simulink model "svpwm_v3"  (R2017a)
settings: Solver=FixedStepAuto  StartTime=0  StopTime=100e-3  FixedStep=1/252000  MaxStep=1e-4  RelTol=1e-4
values from neighbouring files (symbols this model uses):
  Amp = 600    [svpwm_param_v1.m]
  fs = 4e3    (= 4000)    [svpwm_param_v1.m]
  Ts = (1/fs)    (= 0.00025)    [svpwm_param_v1.m]
  Vdc = 700    [svpwm_param_v1.m]
  Vref = 400    [svpwm_param_v1.m]
libraries: powerlib x16, simulink x2, simulink_extras x1
settings Model: Creator=Shuvangkar  LastModifiedBy=Shuvangkar

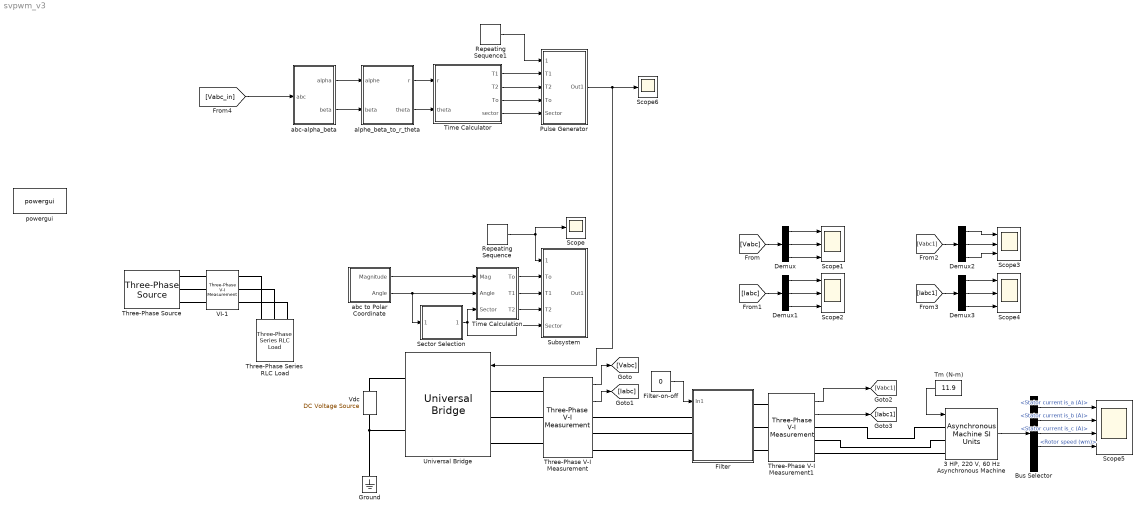
== system svpwm_v3 ==
  "3 HP, 220 V, 60 Hz Asynchronous Machine" : powerlib/Machines/Asynchronous Machine SI Units  RotorType=Squirrel-cage  PresetModel=No  MechanicalLoad=Torque Tm  ShowDetailedParameters=on  ReferenceFrame=Stationary  Units=SI  MeasurementBus=off  NominalParameters=[ 3*746, 220, 60 ]  Stator="[ 0.435  2*2.0e-3 ]"  Rotor="[ 0.816  2.0e-3 ]"  Cage1=[ 0.022 0.226/377]  Cage2=[ 0.022 0.226/377]  Lm=69.31e-3  Mechanical="[ 0.089  0  2 ]"  PolePairs=2  InitialConditions=[0.044533 0 11.138 11.138 11.138 -39.6 -159.6 80.4]  SimulateSaturation=off  Saturation=[0 0;0 0]  LoadFlowParameters=2000  TsPowergui=0  TsBlock=-1  IterativeModel=Trapezoidal non iterative  IterativeDiscreteModel=Trapezoidal non iterative  Pmec=0
  Bus Selector : BusSelector  OutputSignals=Stator measurements.Stator current is_a (A),Stator measurements.Stator current is_b (A),Stator measurements.Stator current is_c (A),Mechanical.Rotor speed (wm),Mechanical.Electromagnetic torque Te (N*m)
  Demux{,1..3} (4 alike) : Demux  Outputs=3
  Filter : Subsystem
  Filter-on-off : Constant  Value=0
  Ground : powerlib/Elements/Ground  LConnTagsString=a
  Pulse Generator : Subsystem
  Repeating Sequence : simulink/Sources/Repeating Sequence  rep_seq_t=[0 1/2 1]*(1/fs)  rep_seq_y=[0 1 0]
  Repeating Sequence1 : simulink/Sources/Repeating Sequence  rep_seq_t=[0 1/2 1]*(1/fs)  rep_seq_y=[0 1 0]
  Scope : Scope
  Scope{1..4} (4 alike) : Scope  NumInputPorts=3
  Scope5 : Scope  NumInputPorts=4
  Scope6 : Scope
  Sector Selection : Subsystem
  Subsystem : Subsystem
  Three-Phase Series RLC Load : powerlib/Elements/Three-Phase Series RLC Load  LConnTagsString=A|B|C  Configuration=Y (grounded)  NominalVoltage=400  Vabc=[1e3 1e3 1e3]  Vabcp=[1e3 1e3 1e3]  NominalFrequency=50  UnbalancedPower=off  ActivePower=10e3  InductivePower=100  CapacitivePower=100  Pabc=[10e3 9e3 11e3]  QLabc=[100 90 110]  QCabc=[100 90 110]  Pabcp=[10e3 9e3 11e3]  QLabcp=[100 90 110]  QCabcp=[100 90 110]  Measurements=None  LoadType=constant Z
  Three-Phase V-I Measurement : powerlib/Measurements/Three-Phase V-I Measurement  VoltageMeasurement=phase-to-phase  SetLabelV=off  LabelV=Vabc  Vpu=off  VpuLL=off  CurrentMeasurement=yes  SetLabelI=off  LabelI=Iabc  Ipu=off  Pbase=100e6  Vbase=500e3  OutputType=Complex  PhasorSimulation=off  PSBequivalent=0
  Three-Phase V-I Measurement1 : powerlib/Measurements/Three-Phase V-I Measurement  VoltageMeasurement=phase-to-ground  SetLabelV=off  LabelV=Vabc  Vpu=off  VpuLL=off  CurrentMeasurement=yes  SetLabelI=off  LabelI=Iabc  Ipu=off  Pbase=100e6  Vbase=500e3  OutputType=Complex  PhasorSimulation=off  PSBequivalent=0
  Three-Phase Source : powerlib/Electrical Sources/Three-Phase Source  InternalConnection=Yg  VoltagePhases=off  Voltage=400  PhaseAngle=0  Voltage_phases=[25e3 25e3 25e3]/sqrt(3)  PhaseAngles_phases=[0 -120 +120]  Frequency=50  NonIdealSource=on  SpecifyImpedance=off  Resistance=0.8929  Inductance=16.58e-3  ShortCircuitLevel=100e6  BaseVoltage=25e3  XRratio=7  BusType=swing  Pref=10e3  Qref=0  Prefabc=[10e3, 10e3, 10e3]  Qrefabc=[0, 0, 0]  Qmin=-inf  Qmax=inf
  Time Calculation : Subsystem
  Time Calculator : Subsystem
  Tm (N-m) : Constant  Value=11.9
  Universal Bridge : powerlib/Power Electronics/Universal Bridge  Arms=3  SnubberResistance=1e5  SnubberCapacitance=inf  Device=MOSFET / Diodes  Ron=1e-3  Lon=0  ForwardVoltages="[  0  0  ]"  ForwardVoltage=0  GTOparameters=[ 10e-6 , 20e-6 ]  IGBTparameters=[ 1e-6 , 2e-6 ]  Measurements=None  Measurements_2=None  converterType=Rectifier
  VI-1 : powerlib/Measurements/Three-Phase V-I Measurement  VoltageMeasurement=phase-to-ground  SetLabelV=on  LabelV=Vabc_in  Vpu=off  VpuLL=off  CurrentMeasurement=yes  SetLabelI=on  LabelI=Iabc_in  Ipu=off  Pbase=100e6  Vbase=500e3  OutputType=Complex  PhasorSimulation=off  PSBequivalent=0
  Vdc : powerlib/Electrical Sources/DC Voltage Source  Amplitude=Amp  Measurements=None
  abc to Polar Coordinate : Subsystem
  abc-alpha_beta : Subsystem
  alphe_beta_to_r_theta : Subsystem
  powergui : powerlib/powergui  Priority=1  SimulationMode=Discrete  SampleTime=1/252000  frequency=60  Iterations=50  frequencyindice=60  Pbase=100e6  ErrMax=1e-4  UnitsV=kV  UnitsW=MW  buscounter=0  FunctionMessages=off  echomessages=off  EnableUseOfTLC=off  CurrentSourceSwitches=off  DisableSnubberDevices=off  DisableRonSwitches=off  DisableVfSwitches=off  DisplayEquations=off  SolverType=Tustin/Backward Euler (TBE)  Interpol=off  ExternalGateDelay=off  methode=off  Ts=100  x0status=blocks  SPID=off  SwTol=0  HookPort=off  RestoreLinks=warning  ResistiveCurrentMeasurement=off  Frange=[0:2:500]  Ylog=off  Xlog=on  ShowGrid=off  save=off  variable=ZData  structure=0  ZoomFFT=off  StartTime=0.0  cycles=1  DisplayStyle=1  fundamental=60  FreqAxis=off  MaxFrequency=1000  frequencyindicesteady=1  RmsSteady=1  display=off
  wires:
  abc to Polar Coordinate/2(Angle) -> Sector Selection/1(Angle), Time Calculation/2(Angle)
  abc to Polar Coordinate/1(Magnitude) -> Time Calculation/1(Mag)
  Sector Selection/1(Sector) -> Subsystem/5(Sector), Time Calculation/3(Sector)
  Repeating Sequence/1 -> Scope/1, Subsystem/1(Sequence)
  Time Calculation/1(To) -> Subsystem/2(To)
  Time Calculation/3(T2) -> Subsystem/4(T2)
  Time Calculation/2(T1) -> Subsystem/3(T1)
  Filter-on-off/1 -> Filter/1(In1)
  Three-Phase V-I Measurement/1 -> [Vabc]
  Three-Phase V-I Measurement/2 -> [Iabc]
  [Vabc] -> Demux/1
  Demux/1 -> Scope1/1
  Demux/2 -> Scope1/2
  Demux/3 -> Scope1/3
  Demux1/2 -> Scope2/2
  [Iabc] -> Demux1/1
  Demux1/1 -> Scope2/1
  Demux1/3 -> Scope2/3
  Three-Phase V-I Measurement1/2 -> [Iabc1]
  Three-Phase V-I Measurement1/1 -> [Vabc1]
  [Iabc1] -> Demux3/1
  Demux2/3 -> Scope3/3
  Demux3/3 -> Scope4/3
  Demux2/2 -> Scope3/2
  Demux2/1 -> Scope3/1
  [Vabc1] -> Demux2/1
  Demux3/2 -> Scope4/2
  Demux3/1 -> Scope4/1
  Tm (N-m)/1 -> "3 HP, 220 V, 60 Hz Asynchronous Machine"/1
  "3 HP, 220 V, 60 Hz Asynchronous Machine"/1 -> Bus Selector/1
  Bus Selector/1 -> Scope5/1  "<Stator current is_a (A)>"
  Bus Selector/2 -> Scope5/2  "<Stator current is_b (A)>"
  Bus Selector/3 -> Scope5/3  "<Stator current is_c (A)>"
  Bus Selector/4 -> Scope5/4  "<Rotor speed (wm)>"
  [Vabc_in] -> abc-alpha_beta/1(abc)
  abc-alpha_beta/1(alpha) -> alphe_beta_to_r_theta/1(alphe)
  abc-alpha_beta/2(beta) -> alphe_beta_to_r_theta/2(beta)
  alphe_beta_to_r_theta/1(r) -> Time Calculator/1(r)
  alphe_beta_to_r_theta/2(theta) -> Time Calculator/2(theta)
  Repeating Sequence1/1 -> Pulse Generator/1(Sequence)
  Pulse Generator/1(Out1) -> Universal Bridge/1, Scope6/1
  Time Calculator/1(T1) -> Pulse Generator/2(T1)
  Time Calculator/2(T2) -> Pulse Generator/3(T2)
  Time Calculator/3(To) -> Pulse Generator/4(To)
  Time Calculator/4(sector) -> Pulse Generator/5(Sector)
  connections:
  Universal Bridge/RConn2 -- Vdc/LConn1 -- Ground/LConn1
  Vdc/RConn1 -- Universal Bridge/RConn1
  Three-Phase V-I Measurement/LConn1 -- Universal Bridge/LConn1
  Three-Phase V-I Measurement/LConn2 -- Universal Bridge/LConn2
  Three-Phase V-I Measurement/LConn3 -- Universal Bridge/LConn3
  Three-Phase V-I Measurement/RConn1 -- Filter/LConn1
  Three-Phase V-I Measurement/RConn2 -- Filter/LConn2
  Three-Phase V-I Measurement/RConn3 -- Filter/LConn3
  Filter/RConn1 -- Three-Phase V-I Measurement1/LConn1
  Filter/RConn2 -- Three-Phase V-I Measurement1/LConn2
  Filter/RConn3 -- Three-Phase V-I Measurement1/LConn3
  "3 HP, 220 V, 60 Hz Asynchronous Machine"/LConn1 -- Three-Phase V-I Measurement1/RConn1
  "3 HP, 220 V, 60 Hz Asynchronous Machine"/LConn2 -- Three-Phase V-I Measurement1/RConn2
  "3 HP, 220 V, 60 Hz Asynchronous Machine"/LConn3 -- Three-Phase V-I Measurement1/RConn3
  VI-1/LConn1 -- Three-Phase Source/RConn1
  VI-1/LConn2 -- Three-Phase Source/RConn2
  VI-1/LConn3 -- Three-Phase Source/RConn3
  VI-1/RConn1 -- Three-Phase Series RLC Load/LConn1
  VI-1/RConn2 -- Three-Phase Series RLC Load/LConn2
  VI-1/RConn3 -- Three-Phase Series RLC Load/LConn3

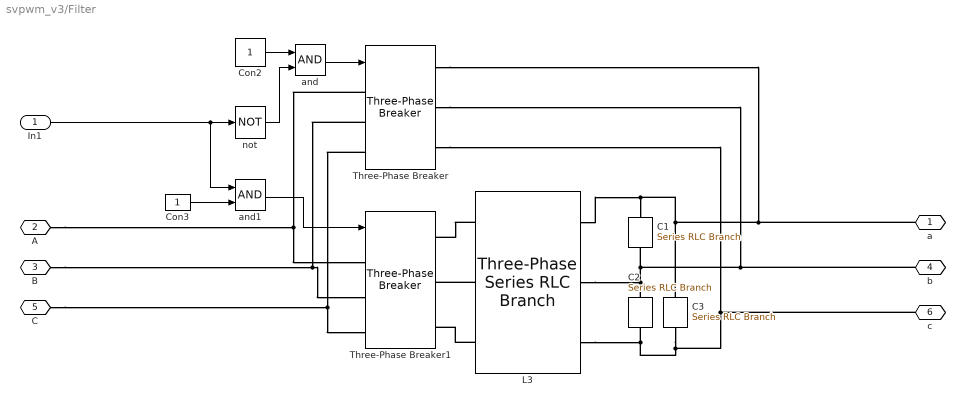
== system svpwm_v3/Filter ==
  In1 : Inport
  C1 : powerlib/Elements/Series RLC Branch  LConnTagsString=__new0  RConnTagsString=__new0  BranchType=C  Resistance=1  Inductance=1e-3  SetiL0=off  InitialCurrent=0  Capacitance=5e-6  Setx0=off  InitialVoltage=0  Measurements=None
  C2 : powerlib/Elements/Series RLC Branch  LConnTagsString=__new0  RConnTagsString=__new0  BranchType=C  Resistance=1  Inductance=1e-3  SetiL0=off  InitialCurrent=0  Capacitance=5e-6  Setx0=off  InitialVoltage=0  Measurements=None
  C3 : powerlib/Elements/Series RLC Branch  LConnTagsString=__new0  RConnTagsString=__new0  BranchType=C  Resistance=1  Inductance=1e-3  SetiL0=off  InitialCurrent=0  Capacitance=5e-6  Setx0=off  InitialVoltage=0  Measurements=None
  Con2 : Constant
  Con3 : Constant
  L3 : powerlib/Elements/Three-Phase Series RLC Branch  LConnTagsString=A|B|C  RConnTagsString=A|B|C  BranchType=L  Resistance=1  Inductance=10e-3  Capacitance=1e-6  Measurements=None
  Three-Phase Breaker : powerlib/Elements/Three-Phase Breaker  InitialState=open  SwitchA=on  SwitchB=on  SwitchC=on  SwitchTimes="[1/60  5/60]"  External=on  BreakerResistance=1e-6  SnubberResistance=1e6  SnubberCapacitance=inf  Measurements=None
  Three-Phase Breaker1 : powerlib/Elements/Three-Phase Breaker  InitialState=open  SwitchA=on  SwitchB=on  SwitchC=on  SwitchTimes="[1/60  5/60]"  External=on  BreakerResistance=0.01  SnubberResistance=1e6  SnubberCapacitance=inf  Measurements=None
  and : Logic  AllPortsSameDT=off  OutDataTypeStr=boolean
  and1 : Logic  AllPortsSameDT=off  OutDataTypeStr=boolean
  not : Logic  Operator=NOT  AllPortsSameDT=off  OutDataTypeStr=boolean
  a : PMIOPort  Port=1  Side=Right
  A : PMIOPort  Port=2  Side=Left
  B : PMIOPort  Port=3  Side=Left
  b : PMIOPort  Port=4  Side=Right
  C : PMIOPort  Port=5  Side=Left
  c : PMIOPort  Port=6  Side=Right
  wires:
  Con3/1 -> and1/2
  and/1 -> Three-Phase Breaker/1
  and1/1 -> Three-Phase Breaker1/1
  Con2/1 -> and/1
  In1/1 -> and1/1, not/1
  not/1 -> and/2
  connections:
  Three-Phase Breaker/LConn2 -- B/RConn1 -- Three-Phase Breaker1/LConn2
  L3/LConn1 -- Three-Phase Breaker1/RConn1
  L3/LConn2 -- Three-Phase Breaker1/RConn2
  L3/LConn3 -- Three-Phase Breaker1/RConn3
  Three-Phase Breaker/LConn1 -- A/RConn1 -- Three-Phase Breaker1/LConn1
  L3/RConn2 -- b/RConn1 -- Three-Phase Breaker/RConn2 -- C1/RConn1 -- C2/LConn1
  L3/RConn3 -- c/RConn1 -- Three-Phase Breaker/RConn3 -- C3/LConn1 -- C2/RConn1
  Three-Phase Breaker/LConn3 -- C/RConn1 -- Three-Phase Breaker1/LConn3
  C3/RConn1 -- a/RConn1 -- Three-Phase Breaker/RConn1 -- C1/LConn1 -- L3/RConn1

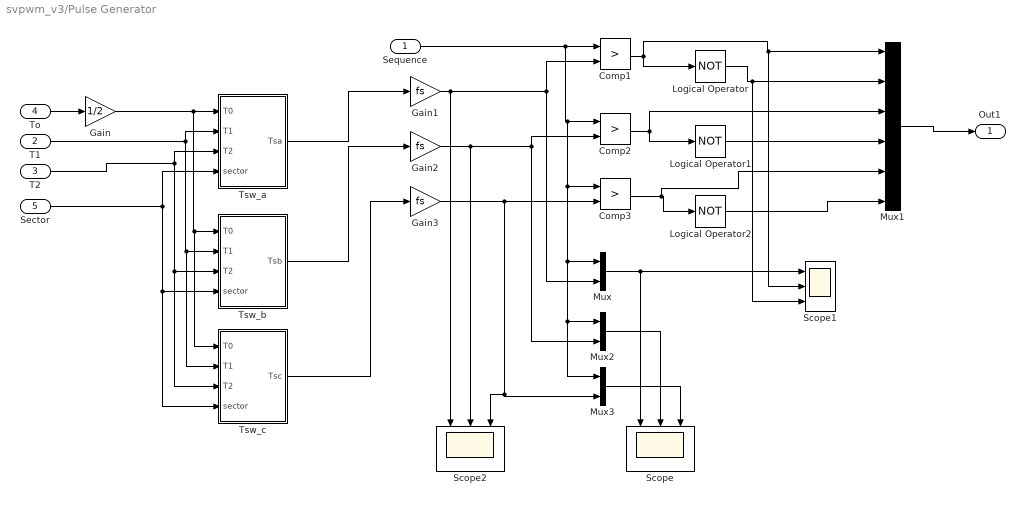
== system svpwm_v3/Pulse Generator ==
  Sequence : Inport
  T1 : Inport  Port=2
  T2 : Inport  Port=3
  To : Inport  Port=4
  Sector : Inport  Port=5
  Comp1 : RelationalOperator  Operator=>  OutDataTypeStr=boolean  RndMeth=Simplest
  Comp2 : RelationalOperator  Operator=>  OutDataTypeStr=boolean  RndMeth=Simplest
  Comp3 : RelationalOperator  Operator=>  OutDataTypeStr=boolean  RndMeth=Simplest
  Gain : Gain  Gain=1/2
  Gain1 : Gain  Gain=fs
  Gain2 : Gain  Gain=fs
  Gain3 : Gain  Gain=fs
  Logical Operator : Logic  Operator=NOT  AllPortsSameDT=off  OutDataTypeStr=boolean
  Logical Operator1 : Logic  Operator=NOT  AllPortsSameDT=off  OutDataTypeStr=boolean
  Logical Operator2 : Logic  Operator=NOT  AllPortsSameDT=off  OutDataTypeStr=boolean
  Mux : Mux  Inputs=2
  Mux1 : Mux  Inputs=6
  Mux2 : Mux  Inputs=2
  Mux3 : Mux  Inputs=2
  Scope : Scope  NumInputPorts=3
  Scope1 : Scope  NumInputPorts=3
  Scope2 : Scope  NumInputPorts=3
  Tsw_a : MATLAB Function  TreatAsAtomicUnit=on
  Tsw_b : MATLAB Function  TreatAsAtomicUnit=on
  Tsw_c : MATLAB Function  TreatAsAtomicUnit=on
  Out1 : Outport
  wires:
  Sector/1 -> Tsw_c/4(sector), Tsw_b/4(sector), Tsw_a/4(sector)
  To/1 -> Gain/1
  Gain/1 -> Tsw_c/1(T0), Tsw_b/1(T0), Tsw_a/1(T0)
  T2/1 -> Tsw_c/3(T2), Tsw_b/3(T2), Tsw_a/3(T2)
  T1/1 -> Tsw_c/2(T1), Tsw_b/2(T1), Tsw_a/2(T1)
  Mux1/1 -> Out1/1
  Gain2/1 -> Scope2/2, Mux2/2, Comp2/2
  Logical Operator2/1 -> Mux1/6
  Gain3/1 -> Scope2/3, Mux3/2, Comp3/2
  Comp1/1 -> Logical Operator/1, Scope1/2, Mux1/1
  Comp3/1 -> Mux1/5, Logical Operator2/1
  Sequence/1 -> Mux3/1, Mux2/1, Mux/1, Comp3/1, Comp2/1, Comp1/1
  Comp2/1 -> Logical Operator1/1, Mux1/3
  Logical Operator/1 -> Scope1/3, Mux1/2
  Logical Operator1/1 -> Mux1/4
  Gain1/1 -> Scope2/1, Mux/2, Comp1/2
  Tsw_a/1(Tsa) -> Gain1/1
  Tsw_b/1(Tsb) -> Gain2/1
  Tsw_c/1(Tsc) -> Gain3/1
  Mux2/1 -> Scope/2
  Mux/1 -> Scope1/1, Scope/1
  Mux3/1 -> Scope/3

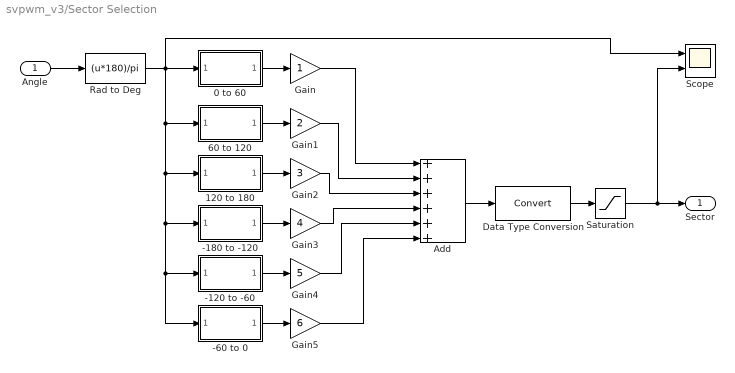
== system svpwm_v3/Sector Selection ==
  Angle : Inport
  -120 to -60 : Subsystem
  -180 to -120 : Subsystem
  -60 to 0 : Subsystem
  0 to 60 : Subsystem
  120 to 180 : Subsystem
  60 to 120 : Subsystem
  Add : Sum  Inputs=++++++
  Data Type Conversion : DataTypeConversion
  Gain : Gain
  Gain1 : Gain  Gain=2
  Gain2 : Gain  Gain=3
  Gain3 : Gain  Gain=4
  Gain4 : Gain  Gain=5
  Gain5 : Gain  Gain=6
  Rad to Deg : Fcn  Expr=(u*180)/pi
  Saturation : Saturate  UpperLimit=6  LowerLimit=1
  Scope : Scope  NumInputPorts=2
  Sector : Outport
  wires:
  Rad to Deg/1 -> Scope/1, -120 to -60/1(Angle), -60 to 0/1(Angle), -180 to -120/1(Angle), 120 to 180/1(Angle), 60 to 120/1(Angle), 0 to 60/1(Angle)
  Angle/1 -> Rad to Deg/1
  Gain4/1 -> Add/5
  0 to 60/1(sector) -> Gain/1
  60 to 120/1(sector) -> Gain1/1
  -120 to -60/1(sector) -> Gain4/1
  -180 to -120/1(sector) -> Gain3/1
  Gain5/1 -> Add/6
  -60 to 0/1(sector) -> Gain5/1
  Gain/1 -> Add/1
  120 to 180/1(sector) -> Gain2/1
  Gain1/1 -> Add/2
  Gain2/1 -> Add/3
  Gain3/1 -> Add/4
  Saturation/1 -> Scope/2, Sector/1
  Add/1 -> Data Type Conversion/1
  Data Type Conversion/1 -> Saturation/1

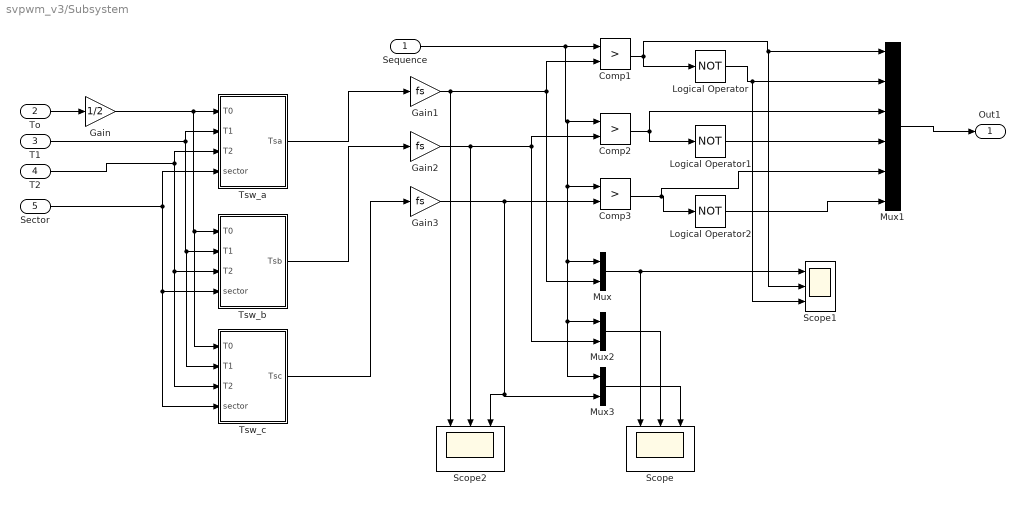
== system svpwm_v3/Subsystem ==
  Sequence : Inport
  To : Inport  Port=2
  T1 : Inport  Port=3
  T2 : Inport  Port=4
  Sector : Inport  Port=5
  Comp1 : RelationalOperator  Operator=>  OutDataTypeStr=boolean  RndMeth=Simplest
  Comp2 : RelationalOperator  Operator=>  OutDataTypeStr=boolean  RndMeth=Simplest
  Comp3 : RelationalOperator  Operator=>  OutDataTypeStr=boolean  RndMeth=Simplest
  Gain : Gain  Gain=1/2
  Gain1 : Gain  Gain=fs
  Gain2 : Gain  Gain=fs
  Gain3 : Gain  Gain=fs
  Logical Operator : Logic  Operator=NOT  AllPortsSameDT=off  OutDataTypeStr=boolean
  Logical Operator1 : Logic  Operator=NOT  AllPortsSameDT=off  OutDataTypeStr=boolean
  Logical Operator2 : Logic  Operator=NOT  AllPortsSameDT=off  OutDataTypeStr=boolean
  Mux : Mux  Inputs=2
  Mux1 : Mux  Inputs=6
  Mux2 : Mux  Inputs=2
  Mux3 : Mux  Inputs=2
  Scope : Scope  NumInputPorts=3
  Scope1 : Scope  NumInputPorts=3
  Scope2 : Scope  NumInputPorts=3
  Tsw_a : MATLAB Function  TreatAsAtomicUnit=on
  Tsw_b : MATLAB Function  TreatAsAtomicUnit=on
  Tsw_c : MATLAB Function  TreatAsAtomicUnit=on
  Out1 : Outport
  wires:
  Sector/1 -> Tsw_c/4(sector), Tsw_b/4(sector), Tsw_a/4(sector)
  To/1 -> Gain/1
  Gain/1 -> Tsw_c/1(T0), Tsw_b/1(T0), Tsw_a/1(T0)
  T2/1 -> Tsw_c/3(T2), Tsw_b/3(T2), Tsw_a/3(T2)
  T1/1 -> Tsw_c/2(T1), Tsw_b/2(T1), Tsw_a/2(T1)
  Mux1/1 -> Out1/1
  Gain2/1 -> Scope2/2, Mux2/2, Comp2/2
  Logical Operator2/1 -> Mux1/6
  Gain3/1 -> Scope2/3, Mux3/2, Comp3/2
  Comp1/1 -> Logical Operator/1, Scope1/2, Mux1/1
  Comp3/1 -> Mux1/5, Logical Operator2/1
  Sequence/1 -> Mux3/1, Mux2/1, Mux/1, Comp3/1, Comp2/1, Comp1/1
  Comp2/1 -> Logical Operator1/1, Mux1/3
  Logical Operator/1 -> Scope1/3, Mux1/2
  Logical Operator1/1 -> Mux1/4
  Gain1/1 -> Scope2/1, Mux/2, Comp1/2
  Tsw_a/1(Tsa) -> Gain1/1
  Tsw_b/1(Tsb) -> Gain2/1
  Tsw_c/1(Tsc) -> Gain3/1
  Mux2/1 -> Scope/2
  Mux/1 -> Scope1/1, Scope/1
  Mux3/1 -> Scope/3

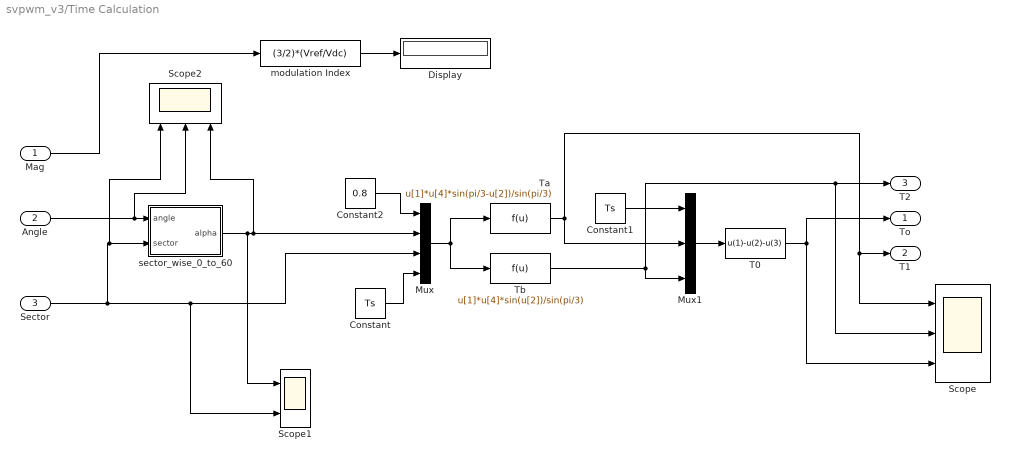
== system svpwm_v3/Time Calculation ==
  Mag : Inport
  Angle : Inport  Port=2
  Sector : Inport  Port=3
  Constant : Constant  Value=Ts
  Constant1 : Constant  Value=Ts
  Constant2 : Constant  Value=0.8
  Display : Display
  Mux : Mux
  Mux1 : Mux  Inputs=3
  Scope : Scope  NumInputPorts=3
  Scope1 : Scope  NumInputPorts=2
  Scope2 : Scope  NumInputPorts=3
  T0 : Fcn  Expr=u(1)-u(2)-u(3)
  Ta : Fcn  Expr=u[1]*u[4]*sin(pi/3-u[2])/sin(pi/3)
  Tb : Fcn  Expr=u[1]*u[4]*sin(u[2])/sin(pi/3)
  modulation Index : Fcn  Expr=(3/2)*(Vref/Vdc)
  "sector_wise_0_to_60 " : MATLAB Function  TreatAsAtomicUnit=on
  To : Outport
  T1 : Outport  Port=2
  T2 : Outport  Port=3
  wires:
  Mux1/1 -> T0/1
  modulation Index/1 -> Display/1
  Constant/1 -> Mux/4
  Ta/1 -> Scope/1, T1/1, Mux1/2
  T0/1 -> Scope/3, To/1
  Tb/1 -> Scope/2, T2/1, Mux1/3
  Mux/1 -> Tb/1, Ta/1
  Sector/1 -> Scope2/1, "sector_wise_0_to_60 "/2(sector), Scope1/2, Mux/3
  Constant1/1 -> Mux1/1
  Mag/1 -> modulation Index/1
  Constant2/1 -> Mux/1
  "sector_wise_0_to_60 "/1(alpha) -> Scope1/1, Scope2/3, Mux/2
  Angle/1 -> Scope2/2, "sector_wise_0_to_60 "/1(angle)

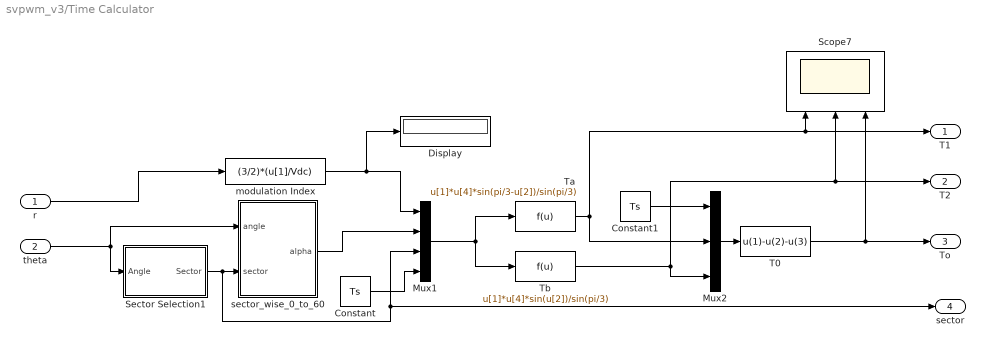
== system svpwm_v3/Time Calculator ==
  r : Inport
  theta : Inport  Port=2
  Constant : Constant  Value=Ts
  Constant1 : Constant  Value=Ts
  Display : Display
  Mux1 : Mux
  Mux2 : Mux  Inputs=3
  Scope7 : Scope  NumInputPorts=3
  Sector Selection1 : Subsystem
  T0 : Fcn  Expr=u(1)-u(2)-u(3)
  Ta : Fcn  Expr=u[1]*u[4]*sin(pi/3-u[2])/sin(pi/3)
  Tb : Fcn  Expr=u[1]*u[4]*sin(u[2])/sin(pi/3)
  modulation Index : Fcn  Expr=(3/2)*(u[1]/Vdc)
  "sector_wise_0_to_60 " : MATLAB Function  TreatAsAtomicUnit=on
  T1 : Outport
  T2 : Outport  Port=2
  To : Outport  Port=3
  sector : Outport  Port=4
  wires:
  Sector Selection1/1(Sector) -> sector/1, Mux1/3, "sector_wise_0_to_60 "/2(sector)
  r/1 -> modulation Index/1
  theta/1 -> Sector Selection1/1(Angle), "sector_wise_0_to_60 "/1(angle)
  modulation Index/1 -> Display/1, Mux1/1
  Constant1/1 -> Mux2/1
  Tb/1 -> T2/1, Scope7/2, Mux2/3
  Ta/1 -> T1/1, Scope7/1, Mux2/2
  Mux1/1 -> Tb/1, Ta/1
  Mux2/1 -> T0/1
  Constant/1 -> Mux1/4
  T0/1 -> To/1, Scope7/3
  "sector_wise_0_to_60 "/1(alpha) -> Mux1/2

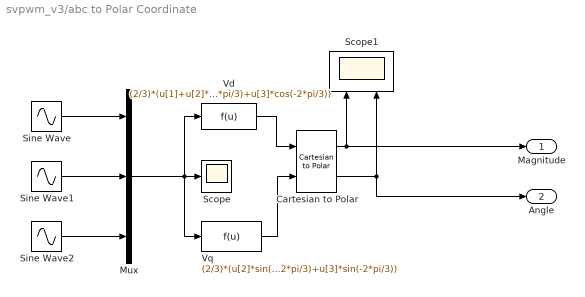
== system svpwm_v3/abc to Polar Coordinate ==
  Cartesian to Polar : simulink_extras/Transformations/Cartesian to Polar
      settings: SourceProductName=Simulink
  Mux : Mux  Inputs=3
  Scope : Scope
  Scope1 : Scope  NumInputPorts=2
  Sine Wave : Sin  Amplitude=Amp  Frequency=2*pi*50  SampleTime=0
  Sine Wave1 : Sin  Amplitude=Amp  Frequency=2*pi*50  Phase=2*pi/3  SampleTime=0
  Sine Wave2 : Sin  Amplitude=Amp  Frequency=2*pi*50  Phase=4*pi/3  SampleTime=0
  Vd : Fcn  Expr=(2/3)*(u[1]+u[2]*cos(2*pi/3)+u[3]*cos(-2*pi/3))
  Vq : Fcn  Expr=(2/3)*(u[2]*sin(2*pi/3)+u[3]*sin(-2*pi/3))
  Magnitude : Outport
  Angle : Outport  Port=2
  wires:
  Mux/1 -> Vq/1, Vd/1, Scope/1
  Cartesian to Polar/2 -> Angle/1, Scope1/2
  Cartesian to Polar/1 -> Magnitude/1, Scope1/1
  Vq/1 -> Cartesian to Polar/2
  Vd/1 -> Cartesian to Polar/1
  Sine Wave/1 -> Mux/1
  Sine Wave1/1 -> Mux/2
  Sine Wave2/1 -> Mux/3

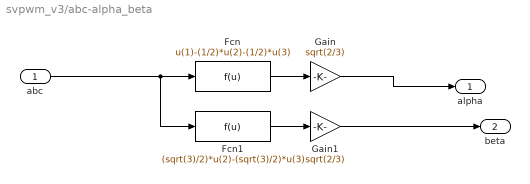
== system svpwm_v3/abc-alpha_beta ==
  abc : Inport
  Fcn : Fcn  Expr=u(1)-(1/2)*u(2)-(1/2)*u(3)
  Fcn1 : Fcn  Expr=(sqrt(3)/2)*u(2)-(sqrt(3)/2)*u(3)
  Gain : Gain  Gain=sqrt(2/3)
  Gain1 : Gain  Gain=sqrt(2/3)
  alpha : Outport
  beta : Outport  Port=2
  wires:
  abc/1 -> Fcn1/1, Fcn/1
  Gain/1 -> alpha/1
  Fcn/1 -> Gain/1
  Fcn1/1 -> Gain1/1
  Gain1/1 -> beta/1

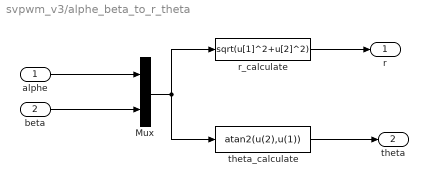
== system svpwm_v3/alphe_beta_to_r_theta ==
  alphe : Inport
  beta : Inport  Port=2
  Mux : Mux  Inputs=2
  r_calculate : Fcn  Expr=sqrt(u[1]^2+u[2]^2)
  theta_calculate : Fcn  Expr=atan2(u(2),u(1))
  r : Outport
  theta : Outport  Port=2
  wires:
  Mux/1 -> theta_calculate/1, r_calculate/1
  theta_calculate/1 -> theta/1
  r_calculate/1 -> r/1
  alphe/1 -> Mux/1
  beta/1 -> Mux/2

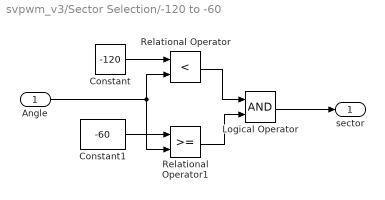
== system svpwm_v3/Sector Selection/-120 to -60 ==
  Angle : Inport
  Constant : Constant  Value=-120
  Constant1 : Constant  Value=-60
  Logical Operator : Logic  AllPortsSameDT=off  OutDataTypeStr=boolean
  Relational Operator : RelationalOperator  Operator=<  OutDataTypeStr=boolean  RndMeth=Simplest
  Relational Operator1 : RelationalOperator  OutDataTypeStr=boolean  RndMeth=Simplest
  sector : Outport
  wires:
  Relational Operator/1 -> Logical Operator/1
  Constant1/1 -> Relational Operator1/1
  Constant/1 -> Relational Operator/1
  Relational Operator1/1 -> Logical Operator/2
  Angle/1 -> Relational Operator/2, Relational Operator1/2
  Logical Operator/1 -> sector/1

== system svpwm_v3/Sector Selection/-180 to -120 ==
  Angle : Inport
  Constant : Constant  Value=-180
  Constant1 : Constant  Value=-120
  Logical Operator : Logic  AllPortsSameDT=off  OutDataTypeStr=boolean
  Relational Operator : RelationalOperator  Operator=<  OutDataTypeStr=boolean  RndMeth=Simplest
  Relational Operator1 : RelationalOperator  OutDataTypeStr=boolean  RndMeth=Simplest
  sector : Outport
  wires:
  Relational Operator/1 -> Logical Operator/1
  Constant1/1 -> Relational Operator1/1
  Constant/1 -> Relational Operator/1
  Relational Operator1/1 -> Logical Operator/2
  Angle/1 -> Relational Operator/2, Relational Operator1/2
  Logical Operator/1 -> sector/1

== system svpwm_v3/Sector Selection/-60 to 0 ==
  Angle : Inport
  Constant : Constant  Value=-60
  Constant1 : Constant  Value=0
  Logical Operator : Logic  AllPortsSameDT=off  OutDataTypeStr=boolean
  Relational Operator : RelationalOperator  Operator=<  OutDataTypeStr=boolean  RndMeth=Simplest
  Relational Operator1 : RelationalOperator  OutDataTypeStr=boolean  RndMeth=Simplest
  sector : Outport
  wires:
  Relational Operator/1 -> Logical Operator/1
  Constant1/1 -> Relational Operator1/1
  Constant/1 -> Relational Operator/1
  Relational Operator1/1 -> Logical Operator/2
  Angle/1 -> Relational Operator/2, Relational Operator1/2
  Logical Operator/1 -> sector/1

== system svpwm_v3/Sector Selection/0 to 60 ==
  Angle : Inport
  Constant : Constant  Value=0
  Constant1 : Constant  Value=60
  Logical Operator : Logic  AllPortsSameDT=off  OutDataTypeStr=boolean
  Relational Operator : RelationalOperator  Operator=<  OutDataTypeStr=boolean  RndMeth=Simplest
  Relational Operator1 : RelationalOperator  OutDataTypeStr=boolean  RndMeth=Simplest
  sector : Outport
  wires:
  Relational Operator/1 -> Logical Operator/1
  Constant1/1 -> Relational Operator1/1
  Constant/1 -> Relational Operator/1
  Relational Operator1/1 -> Logical Operator/2
  Angle/1 -> Relational Operator1/2, Relational Operator/2
  Logical Operator/1 -> sector/1

== system svpwm_v3/Sector Selection/120 to 180 ==
  Angle : Inport
  Constant : Constant  Value=120
  Constant1 : Constant  Value=180
  Logical Operator : Logic  AllPortsSameDT=off  OutDataTypeStr=boolean
  Relational Operator : RelationalOperator  Operator=<  OutDataTypeStr=boolean  RndMeth=Simplest
  Relational Operator1 : RelationalOperator  OutDataTypeStr=boolean  RndMeth=Simplest
  sector : Outport
  wires:
  Relational Operator/1 -> Logical Operator/1
  Constant1/1 -> Relational Operator1/1
  Constant/1 -> Relational Operator/1
  Relational Operator1/1 -> Logical Operator/2
  Angle/1 -> Relational Operator/2, Relational Operator1/2
  Logical Operator/1 -> sector/1

== system svpwm_v3/Sector Selection/60 to 120 ==
  Angle : Inport
  Constant : Constant  Value=60
  Constant1 : Constant  Value=120
  Logical Operator : Logic  AllPortsSameDT=off  OutDataTypeStr=boolean
  Relational Operator : RelationalOperator  Operator=<  OutDataTypeStr=boolean  RndMeth=Simplest
  Relational Operator1 : RelationalOperator  OutDataTypeStr=boolean  RndMeth=Simplest
  sector : Outport
  wires:
  Relational Operator/1 -> Logical Operator/1
  Constant1/1 -> Relational Operator1/1
  Constant/1 -> Relational Operator/1
  Relational Operator1/1 -> Logical Operator/2
  Angle/1 -> Relational Operator/2, Relational Operator1/2
  Logical Operator/1 -> sector/1

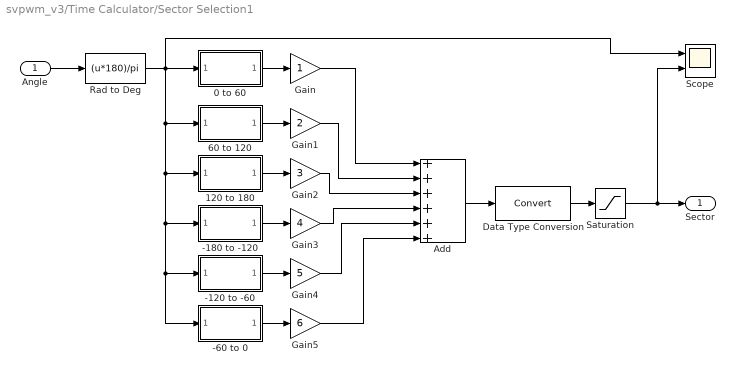
== system svpwm_v3/Time Calculator/Sector Selection1 ==
  Angle : Inport
  -120 to -60 : Subsystem
  -180 to -120 : Subsystem
  -60 to 0 : Subsystem
  0 to 60 : Subsystem
  120 to 180 : Subsystem
  60 to 120 : Subsystem
  Add : Sum  Inputs=++++++
  Data Type Conversion : DataTypeConversion
  Gain : Gain
  Gain1 : Gain  Gain=2
  Gain2 : Gain  Gain=3
  Gain3 : Gain  Gain=4
  Gain4 : Gain  Gain=5
  Gain5 : Gain  Gain=6
  Rad to Deg : Fcn  Expr=(u*180)/pi
  Saturation : Saturate  UpperLimit=6  LowerLimit=1
  Scope : Scope  NumInputPorts=2
  Sector : Outport
  wires:
  Rad to Deg/1 -> Scope/1, -120 to -60/1(Angle), -60 to 0/1(Angle), -180 to -120/1(Angle), 120 to 180/1(Angle), 60 to 120/1(Angle), 0 to 60/1(Angle)
  Angle/1 -> Rad to Deg/1
  Gain4/1 -> Add/5
  0 to 60/1(sector) -> Gain/1
  60 to 120/1(sector) -> Gain1/1
  -120 to -60/1(sector) -> Gain4/1
  -180 to -120/1(sector) -> Gain3/1
  Gain5/1 -> Add/6
  -60 to 0/1(sector) -> Gain5/1
  Gain/1 -> Add/1
  120 to 180/1(sector) -> Gain2/1
  Gain1/1 -> Add/2
  Gain2/1 -> Add/3
  Gain3/1 -> Add/4
  Saturation/1 -> Scope/2, Sector/1
  Add/1 -> Data Type Conversion/1
  Data Type Conversion/1 -> Saturation/1

== system svpwm_v3/Time Calculator/Sector Selection1/-120 to -60 ==
  Angle : Inport
  Constant : Constant  Value=-120
  Constant1 : Constant  Value=-60
  Logical Operator : Logic  AllPortsSameDT=off  OutDataTypeStr=boolean
  Relational Operator : RelationalOperator  Operator=<  OutDataTypeStr=boolean  RndMeth=Simplest
  Relational Operator1 : RelationalOperator  OutDataTypeStr=boolean  RndMeth=Simplest
  sector : Outport
  wires:
  Relational Operator/1 -> Logical Operator/1
  Constant1/1 -> Relational Operator1/1
  Constant/1 -> Relational Operator/1
  Relational Operator1/1 -> Logical Operator/2
  Angle/1 -> Relational Operator/2, Relational Operator1/2
  Logical Operator/1 -> sector/1

== system svpwm_v3/Time Calculator/Sector Selection1/-180 to -120 ==
  Angle : Inport
  Constant : Constant  Value=-180
  Constant1 : Constant  Value=-120
  Logical Operator : Logic  AllPortsSameDT=off  OutDataTypeStr=boolean
  Relational Operator : RelationalOperator  Operator=<  OutDataTypeStr=boolean  RndMeth=Simplest
  Relational Operator1 : RelationalOperator  OutDataTypeStr=boolean  RndMeth=Simplest
  sector : Outport
  wires:
  Relational Operator/1 -> Logical Operator/1
  Constant1/1 -> Relational Operator1/1
  Constant/1 -> Relational Operator/1
  Relational Operator1/1 -> Logical Operator/2
  Angle/1 -> Relational Operator/2, Relational Operator1/2
  Logical Operator/1 -> sector/1

== system svpwm_v3/Time Calculator/Sector Selection1/-60 to 0 ==
  Angle : Inport
  Constant : Constant  Value=-60
  Constant1 : Constant  Value=0
  Logical Operator : Logic  AllPortsSameDT=off  OutDataTypeStr=boolean
  Relational Operator : RelationalOperator  Operator=<  OutDataTypeStr=boolean  RndMeth=Simplest
  Relational Operator1 : RelationalOperator  OutDataTypeStr=boolean  RndMeth=Simplest
  sector : Outport
  wires:
  Relational Operator/1 -> Logical Operator/1
  Constant1/1 -> Relational Operator1/1
  Constant/1 -> Relational Operator/1
  Relational Operator1/1 -> Logical Operator/2
  Angle/1 -> Relational Operator/2, Relational Operator1/2
  Logical Operator/1 -> sector/1

== system svpwm_v3/Time Calculator/Sector Selection1/0 to 60 ==
  Angle : Inport
  Constant : Constant  Value=0
  Constant1 : Constant  Value=60
  Logical Operator : Logic  AllPortsSameDT=off  OutDataTypeStr=boolean
  Relational Operator : RelationalOperator  Operator=<  OutDataTypeStr=boolean  RndMeth=Simplest
  Relational Operator1 : RelationalOperator  OutDataTypeStr=boolean  RndMeth=Simplest
  sector : Outport
  wires:
  Relational Operator/1 -> Logical Operator/1
  Constant1/1 -> Relational Operator1/1
  Constant/1 -> Relational Operator/1
  Relational Operator1/1 -> Logical Operator/2
  Angle/1 -> Relational Operator1/2, Relational Operator/2
  Logical Operator/1 -> sector/1

== system svpwm_v3/Time Calculator/Sector Selection1/120 to 180 ==
  Angle : Inport
  Constant : Constant  Value=120
  Constant1 : Constant  Value=180
  Logical Operator : Logic  AllPortsSameDT=off  OutDataTypeStr=boolean
  Relational Operator : RelationalOperator  Operator=<  OutDataTypeStr=boolean  RndMeth=Simplest
  Relational Operator1 : RelationalOperator  OutDataTypeStr=boolean  RndMeth=Simplest
  sector : Outport
  wires:
  Relational Operator/1 -> Logical Operator/1
  Constant1/1 -> Relational Operator1/1
  Constant/1 -> Relational Operator/1
  Relational Operator1/1 -> Logical Operator/2
  Angle/1 -> Relational Operator/2, Relational Operator1/2
  Logical Operator/1 -> sector/1

== system svpwm_v3/Time Calculator/Sector Selection1/60 to 120 ==
  Angle : Inport
  Constant : Constant  Value=60
  Constant1 : Constant  Value=120
  Logical Operator : Logic  AllPortsSameDT=off  OutDataTypeStr=boolean
  Relational Operator : RelationalOperator  Operator=<  OutDataTypeStr=boolean  RndMeth=Simplest
  Relational Operator1 : RelationalOperator  OutDataTypeStr=boolean  RndMeth=Simplest
  sector : Outport
  wires:
  Relational Operator/1 -> Logical Operator/1
  Constant1/1 -> Relational Operator1/1
  Constant/1 -> Relational Operator/1
  Relational Operator1/1 -> Logical Operator/2
  Angle/1 -> Relational Operator/2, Relational Operator1/2
  Logical Operator/1 -> sector/1

== matlab function svpwm_v3/Subsystem/Tsw_a ==
  data: T0 input; Tsa output; T1 input; T2 input; sector input
function Tsa = fcn(T0,T1,T2,sector)
if(sector==1)
    Tsa = T0+T1+T2;  
elseif(sector==2)
    Tsa = T1+T0;  
elseif(sector==3)
    Tsa = T0;  
elseif(sector==4)
    Tsa = T0;  
elseif(sector==5)
    Tsa = T2+T0;  
else(sector==6)
    Tsa = T1+T2+T0;
end

== matlab function svpwm_v3/Time Calculation/sector_wise_0_to_60  ==
  data: angle input; alpha output; sector input
function alpha = fcn(angle,sector)
alpha = 0;
if (sector==1)
    alpha = angle;
elseif (sector==2)
    alpha = angle-pi/3;
elseif (sector == 3)
    alpha = angle- (2*pi/3);
elseif (sector==4)
    alpha = angle+pi;
elseif (sector==5)
    alpha = angle+(2*pi/3)
else 
    alpha = angle+pi/3;
end

== matlab function svpwm_v3/Subsystem/Tsw_b ==
  data: T0 input; Tsb output; T1 input; T2 input; sector input
function Tsb = fcn(T0,T1,T2,sector)
if(sector==1)
    Tsb = T2+T0;  
elseif(sector==2)
    Tsb = T0+T1+T2; 
elseif(sector==3)
    Tsb = T0+T1+T2;  
elseif(sector==4)
    Tsb = T0+T1;  
elseif(sector==5)
    Tsb = T0;  
else(sector==6)
    Tsb = T0;
end

== matlab function svpwm_v3/Subsystem/Tsw_c ==
  data: T0 input; Tsc output; T1 input; T2 input; sector input
function Tsc = fcn(T0,T1,T2,sector)
if(sector==1)
    Tsc = T0;  
elseif(sector==2)
    Tsc = T0;  
elseif(sector==3)
    Tsc = T0+T2;  
elseif(sector==4)
    Tsc = T0+T1+T2;  
elseif(sector==5)
    Tsc = T0+T1+T2;  
else(sector==6)
    Tsc = T0+T1;
end

== matlab function svpwm_v3/Time Calculator/sector_wise_0_to_60  ==
  data: angle input; alpha output; sector input
function alpha = fcn(angle,sector)
%This function convert Pi to -Pi into 0 to 60 degree for each sector 
alpha = 0;
if (sector==1)
    alpha = angle;
elseif (sector==2)
    alpha = angle-pi/3;
elseif (sector == 3)
    alpha = angle- (2*pi/3);
elseif (sector==4)
    alpha = angle+pi;
elseif (sector==5)
    alpha = angle+(2*pi/3)
else 
    alpha = angle+pi/3;
end

== matlab function svpwm_v3/Pulse Generator/Tsw_a ==
  data: T0 input; Tsa output; T1 input; T2 input; sector input
function Tsa = fcn(T0,T1,T2,sector)
if(sector==1)
    Tsa = T0+T1+T2;  
elseif(sector==2)
    Tsa = T1+T0;  
elseif(sector==3)
    Tsa = T0;  
elseif(sector==4)
    Tsa = T0;  
elseif(sector==5)
    Tsa = T2+T0;  
else(sector==6)
    Tsa = T1+T2+T0;
end

== matlab function svpwm_v3/Pulse Generator/Tsw_b ==
  data: T0 input; Tsb output; T1 input; T2 input; sector input
function Tsb = fcn(T0,T1,T2,sector)
if(sector==1)
    Tsb = T2+T0;  
elseif(sector==2)
    Tsb = T0+T1+T2; 
elseif(sector==3)
    Tsb = T0+T1+T2;  
elseif(sector==4)
    Tsb = T0+T1;  
elseif(sector==5)
    Tsb = T0;  
else(sector==6)
    Tsb = T0;
end

== matlab function svpwm_v3/Pulse Generator/Tsw_c ==
  data: T0 input; Tsc output; T1 input; T2 input; sector input
function Tsc = fcn(T0,T1,T2,sector)
if(sector==1)
    Tsc = T0;  
elseif(sector==2)
    Tsc = T0;  
elseif(sector==3)
    Tsc = T0+T2;  
elseif(sector==4)
    Tsc = T0+T1+T2;  
elseif(sector==5)
    Tsc = T0+T1+T2;  
else(sector==6)
    Tsc = T0+T1;
end
